simulink model "FOC_HSMO_G474"  (R2020b)
settings: Solver=FixedStepDiscrete  StartTime=0.0  StopTime=10  FixedStep=TsBSP  RelTol=1e-3
PreLoadFcn:
  | a=1;
values from neighbouring files (symbols this model uses):
  BandwidthCurrentPI = 1256.6370614359173    [G474_FOC_HSMO.sldd]
  GainK = 2.0    [G474_FOC_HSMO.sldd]
  GainM = 0.15    [G474_FOC_HSMO.sldd]
  Ld = 0.000195185    [G474_FOC_HSMO.sldd]    (also in Hall_HSMO_FOC_Data.sldd = 0.0004
  Ld_MODEL = 0.000195185    [G474_FOC_HSMO.sldd]
  Lq = 0.000195185    [G474_FOC_HSMO.sldd]    (also in Hall_HSMO_FOC_Data.sldd = 0.00045
  Lq_MODEL = 0.000195185    [G474_FOC_HSMO.sldd]
  MaxVoltage = 10.0    [G474_FOC_HSMO.sldd]
  PolePairs = 5.0    [G474_FOC_HSMO.sldd]
  PolePairs_MODEL = 5.0    [G474_FOC_HSMO.sldd]
  PWMHalfPeriod = 4199.0    [G474_FOC_HSMO.sldd]
  Rs = 0.1764    [G474_FOC_HSMO.sldd]
  TsBSP = 5.0E-6    [G474_FOC_HSMO.sldd]
  TsFOC = 0.0001    [G474_FOC_HSMO.sldd]
  TsFOC_MODEL = 0.0001    [G474_FOC_HSMO.sldd]
undefined symbols (not defined in the file or in its folder): DiscIntNeverNeededParam, sigbuilder_block
libraries: pid_lib x3, mcbplantlib x1, autolibpmsminterior x1
(part 2 of 2)

== system FOC_HSMO_G474/FOC/FOC_CURRENT/HIGH_SMO/QPLL/SpeedToTheta/RangeLimit ==
  In : Inport
  Constant : Constant  Value=2*pi  OutDataTypeStr=single  SampleTime=-1
  Constant1 : Constant  Value=0  OutDataTypeStr=single  SampleTime=-1
  If : If  NumInputs=2  IfExpression=u1  ElseIfExpressions=u2
  If Action Subsystem : Subsystem  TreatAsAtomicUnit=on
  If Action Subsystem1 : Subsystem  TreatAsAtomicUnit=on
  If Action Subsystem2 : Subsystem  TreatAsAtomicUnit=on
  Merge : Merge  Inputs=3
  Relational Operator : RelationalOperator  Operator=>  OutDataTypeStr=boolean  RndMeth=Simplest
  Relational Operator1 : RelationalOperator  Operator=<  OutDataTypeStr=boolean  RndMeth=Simplest
  Theta : Outport
  wires:
  Relational Operator/1 -> If/1
  Constant/1 -> Relational Operator/2
  Constant1/1 -> Relational Operator1/2
  In/1 -> Relational Operator1/1, If Action Subsystem2/1(In1), If Action Subsystem1/1(In1), If Action Subsystem/1(In1), Relational Operator/1
  Relational Operator1/1 -> If/2
  Merge/1 -> Theta/1
  If/3 -> If Action Subsystem2/Action
  If/2 -> If Action Subsystem/Action
  If/1 -> If Action Subsystem1/Action
  If Action Subsystem2/1(Out1) -> Merge/1
  If Action Subsystem/1(Out1) -> Merge/2
  If Action Subsystem1/1(Out1) -> Merge/3

== system FOC_HSMO_G474/FOC/FOC_CURRENT/HIGH_SMO/QPLL/Subsystem1/If Action Subsystem ==
  Action Port : ActionPort  ActionPortLabel=if(u1 > 0)
  Constant : Constant  OutDataTypeStr=single
  Out1 : Outport
  wires:
  Constant/1 -> Out1/1

== system FOC_HSMO_G474/FOC/FOC_CURRENT/HIGH_SMO/QPLL/Subsystem1/If Action Subsystem1 ==
  Action Port : ActionPort  ActionPortLabel=else
  Constant : Constant  Value=-1  OutDataTypeStr=single
  Out1 : Outport
  wires:
  Constant/1 -> Out1/1

== system FOC_HSMO_G474/FOC/FOC_CURRENT/SVPWM/JudgeSector/If Action Subsystem/If Action Subsystem ==
  u_alpha_prime : Inport
  u_beta_prime : Inport  Port=2
  Action Port : ActionPort  ActionPortLabel=if(u1)
  Constant : Constant  Value=2
  Constant1 : Constant
  Gain : Gain  Gain=1/sqrt(3)
  Relational Operator : RelationalOperator  Operator=<  OutDataTypeStr=boolean  RndMeth=Simplest
  Switch : Switch  Criteria=u2 > Threshold
  sector : Outport
  wires:
  u_beta_prime/1 -> Gain/1
  u_alpha_prime/1 -> Relational Operator/1
  Gain/1 -> Relational Operator/2
  Relational Operator/1 -> Switch/2
  Constant/1 -> Switch/1
  Constant1/1 -> Switch/3
  Switch/1 -> sector/1

== system FOC_HSMO_G474/FOC/FOC_CURRENT/SVPWM/JudgeSector/If Action Subsystem/If Action Subsystem1 ==
  u_alpha_prime : Inport
  u_beta_prime : Inport  Port=2
  Action Port : ActionPort  ActionPortLabel=else
  Constant : Constant  Value=3
  Constant1 : Constant  Value=2
  Gain : Gain  Gain=-1/sqrt(3)
  Relational Operator : RelationalOperator  Operator=<  OutDataTypeStr=boolean  RndMeth=Simplest
  Switch : Switch  Criteria=u2 > Threshold
  sector : Outport
  wires:
  u_beta_prime/1 -> Gain/1
  u_alpha_prime/1 -> Relational Operator/1
  Gain/1 -> Relational Operator/2
  Relational Operator/1 -> Switch/2
  Constant/1 -> Switch/1
  Constant1/1 -> Switch/3
  Switch/1 -> sector/1

== system FOC_HSMO_G474/FOC/FOC_CURRENT/SVPWM/JudgeSector/If Action Subsystem1/If Action Subsystem ==
  u_alpha_prime : Inport
  u_beta_prime : Inport  Port=2
  Action Port : ActionPort  ActionPortLabel=if(u1)
  Constant : Constant  Value=5
  Constant1 : Constant  Value=6
  Gain : Gain  Gain=-1/sqrt(3)
  Relational Operator : RelationalOperator  Operator=<  OutDataTypeStr=boolean  RndMeth=Simplest
  Switch : Switch  Criteria=u2 > Threshold
  sector : Outport
  wires:
  u_beta_prime/1 -> Gain/1
  u_alpha_prime/1 -> Relational Operator/1
  Gain/1 -> Relational Operator/2
  Relational Operator/1 -> Switch/2
  Constant/1 -> Switch/1
  Constant1/1 -> Switch/3
  Switch/1 -> sector/1

== system FOC_HSMO_G474/FOC/FOC_CURRENT/SVPWM/JudgeSector/If Action Subsystem1/If Action Subsystem1 ==
  u_alpha_prime : Inport
  u_beta_prime : Inport  Port=2
  Action Port : ActionPort  ActionPortLabel=else
  Constant : Constant  Value=4
  Constant1 : Constant  Value=5
  Gain : Gain  Gain=1/sqrt(3)
  Relational Operator : RelationalOperator  Operator=<  OutDataTypeStr=boolean  RndMeth=Simplest
  Switch : Switch  Criteria=u2 > Threshold
  sector : Outport
  wires:
  u_beta_prime/1 -> Gain/1
  u_alpha_prime/1 -> Relational Operator/1
  Gain/1 -> Relational Operator/2
  Relational Operator/1 -> Switch/2
  Constant/1 -> Switch/1
  Constant1/1 -> Switch/3
  Switch/1 -> sector/1

== system FOC_HSMO_G474/FOC/FOC_CURRENT/HIGH_SMO/QPLL/SpeedToTheta/RangeLimit/If Action Subsystem ==
  In1 : Inport
  Action Port : ActionPort  ActionPortLabel=elseif(u2)
  Constant : Constant  Value=2*pi  OutDataTypeStr=single  SampleTime=-1
  Sum : Sum  Inputs=|++
  Out1 : Outport
  wires:
  In1/1 -> Sum/1
  Constant/1 -> Sum/2
  Sum/1 -> Out1/1

== system FOC_HSMO_G474/FOC/FOC_CURRENT/HIGH_SMO/QPLL/SpeedToTheta/RangeLimit/If Action Subsystem1 ==
  In1 : Inport
  Action Port : ActionPort  ActionPortLabel=if(u1)
  Constant : Constant  Value=2*pi  OutDataTypeStr=single  SampleTime=-1
  Sum : Sum  Inputs=|+-
  Out1 : Outport
  wires:
  In1/1 -> Sum/1
  Constant/1 -> Sum/2
  Sum/1 -> Out1/1

== system FOC_HSMO_G474/FOC/FOC_CURRENT/HIGH_SMO/QPLL/SpeedToTheta/RangeLimit/If Action Subsystem2 ==
  In1 : Inport
  Action Port : ActionPort  ActionPortLabel=else
  Out1 : Outport
  wires:
  In1/1 -> Out1/1
